simulink model "parallel_phase_voltages_per_switching_state_6"  (R2022a)
settings: Solver=FixedStepDiscrete  StartTime=0.0  StopTime=10.0  RelTol=1e-3
values from neighbouring files (symbols this model uses):
  f_c = 100000    [MPC_params.m]
  Rt = 1e-8    (= 1e-08)    [MPC_params.m]
  u_dc = 565    [MPC_params.m]
libraries: simulink x2, hdlsllib x2
(part 1 of 4)
settings Model: DataTypeOverride=Off  Creator=Andre Merx  LastModifiedBy=Andre Merx
settings SolverCC: AlgebraicLoopSolver=TrustRegion
settings DataIOCC: LimitDataPoints=on  SaveOutput=off  SaveTime=off
settings OptimizationCC: BlockReduction=off  ConditionallyExecuteInputs=off  DefaultParameterBehavior=Inlined  LifeSpan=inf
settings DebuggingCC: AlgebraicLoopMsg=error  SingleTaskRateTransMsg=error  UnconnectedInputMsg=warning  UnconnectedOutputMsg=warning  UnconnectedLineMsg=warning  AllowSymbolicDim=off  StrictBusMsg=ErrorOnBusTreatedAsVector  SFUnexpectedBacktrackingDiag=warning  SFNoUnconditionalDefaultTransitionDiag=warning  SFExecutionAtInitializationDiag=none  SFMachineParentedDataDiag=warning  ArithmeticOperatorsInVariantConditions=warning
settings HardwareCC: ProdBitPerPointer=32  ProdBitPerSizeT=32  ProdBitPerPtrDiffT=32  ProdLargestAtomicFloat=None  ProdIntDivRoundTo=Undefined  ProdEndianess=Unspecified  ProdWordSize=32  ProdHWDeviceType=ASIC/FPGA->ASIC/FPGA  ProdEqTarget=off
settings SFSimCC: SimUseLocalCustomCode=off  CustomCodeUndefinedFunction=UseInterfaceOnly
settings RTWCC: RTWUseLocalCustomCode=off
settings CodeAppCC: StateflowObjectComments=on
settings GRTTargetCC: TargetLangStandard=C89/C90 (ANSI)
settings ConfigComp: CovScope=ReferencedModels  CovMetricSettings=dw  CovSaveCumulativeToWorkspaceVar=on  CovSaveSingleToWorkspaceVar=on  CovExternalEMLEnable=off  CovSFcnEnable=off

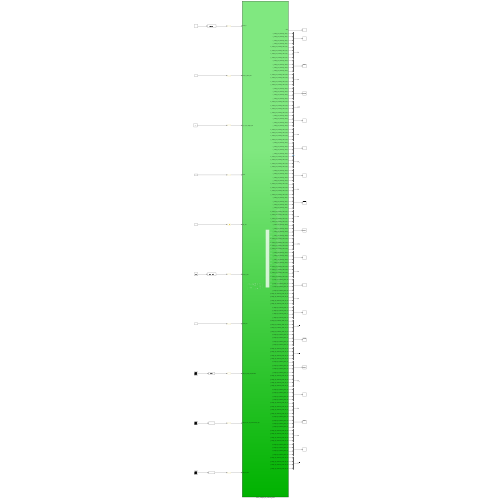
[thumbnail: Simulink's stored preview of the top-level diagram]
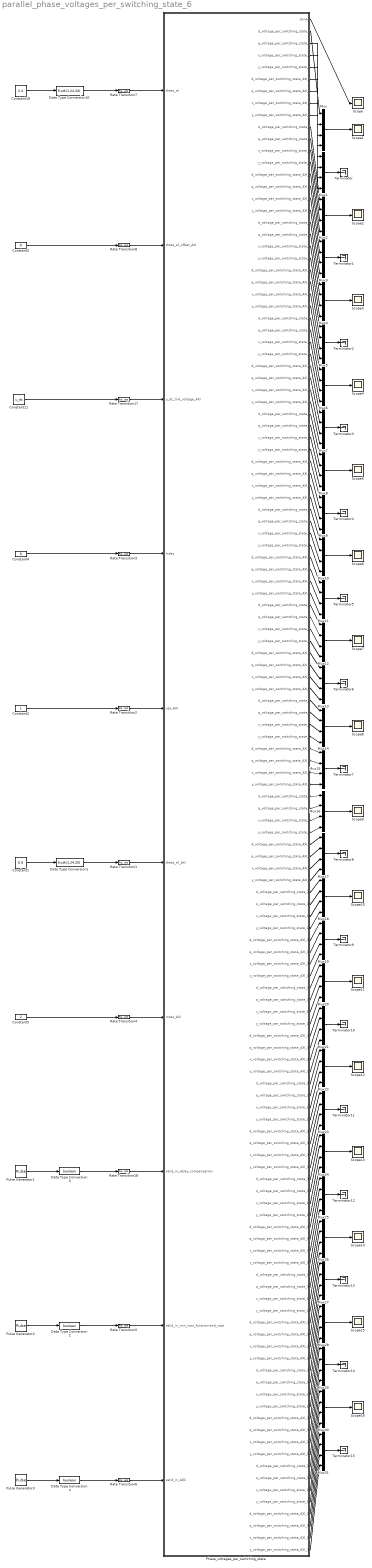
== system parallel_phase_voltages_per_switching_state_6 ==
  Constant1 : Constant  Value=0.9
  Constant11 : Constant  Value=u_dc  OutDataTypeStr=single  SampleTime=-1
  Constant18 : Constant  Value=2.4
  Constant2 : Constant  OutDataTypeStr=boolean  SampleTime=-1
  Constant3 : Constant  Value=0  OutDataTypeStr=single  SampleTime=-1
  Constant4 : Constant  Value=0  OutDataTypeStr=int32  SampleTime=-1
  Constant5 : Constant  Value=2  OutDataTypeStr=int32  SampleTime=-1
  Data Type Conversion1 : DataTypeConversion  OutDataTypeStr=fixdt(1,24,20)  SaturateOnIntegerOverflow=off  RndMeth=Floor
  Data Type Conversion10 : DataTypeConversion  OutDataTypeStr=fixdt(1,24,20)  SaturateOnIntegerOverflow=off  RndMeth=Floor
  Data Type Conversion2 : DataTypeConversion  OutDataTypeStr=boolean  SaturateOnIntegerOverflow=off  RndMeth=Floor
  Data Type Conversion3 : DataTypeConversion  OutDataTypeStr=boolean  SaturateOnIntegerOverflow=off  RndMeth=Floor
  Data Type Conversion4 : DataTypeConversion  OutDataTypeStr=boolean  SaturateOnIntegerOverflow=off  RndMeth=Floor
  Mux{,1..31} (32 alike) : Mux
  Phase_voltages_per_switching_state : Subsystem  TreatAsAtomicUnit=on
  Pulse Generator1 : DiscretePulseGenerator  PulseType=Time based  Period=1/f_c
  Pulse Generator2 : DiscretePulseGenerator  PulseType=Time based  Period=1/f_c
  Pulse Generator3 : DiscretePulseGenerator  PulseType=Time based  Period=1/f_c
  Rate Transition{1..8,17..18} (10 alike) : RateTransition  OutPortSampleTime=Rt
  Scope{,1..16} (17 alike) : Scope
  Terminator{,1..15} (16 alike) : Terminator
  wires:
  Data Type Conversion2/1 -> Rate Transition5/1
  Data Type Conversion3/1 -> Rate Transition18/1
  Rate Transition5/1 -> Phase_voltages_per_switching_state/9(valid_in_min_cost_function-and_vopt)
  Rate Transition4/1 -> Phase_voltages_per_switching_state/7(Index_AXI)
  Constant5/1 -> Rate Transition4/1
  Rate Transition6/1 -> Phase_voltages_per_switching_state/10(valid_in_ADC)
  Data Type Conversion4/1 -> Rate Transition6/1
  Pulse Generator3/1 -> Data Type Conversion4/1
  Pulse Generator2/1 -> Data Type Conversion2/1
  Rate Transition3/1 -> Phase_voltages_per_switching_state/4(Index)
  Data Type Conversion1/1 -> Rate Transition1/1
  Rate Transition18/1 -> Phase_voltages_per_switching_state/8(valid_in_delay_compensation)
  Constant18/1 -> Data Type Conversion10/1
  Rate Transition8/1 -> Phase_voltages_per_switching_state/2(theta_el_offset_AXI)
  Rate Transition1/1 -> Phase_voltages_per_switching_state/6(theta_el_AXI)
  Pulse Generator1/1 -> Data Type Conversion3/1
  Constant1/1 -> Data Type Conversion1/1
  Rate Transition7/1 -> Phase_voltages_per_switching_state/1(theta_el)
  Constant4/1 -> Rate Transition3/1
  Rate Transition17/1 -> Phase_voltages_per_switching_state/3(u_dc_link_voltage_AXI)
  Constant3/1 -> Rate Transition8/1
  Constant11/1 -> Rate Transition17/1
  Constant2/1 -> Rate Transition2/1
  Rate Transition2/1 -> Phase_voltages_per_switching_state/5(use_AXI)
  Data Type Conversion10/1 -> Rate Transition7/1
  Phase_voltages_per_switching_state/1(done) -> Scope/1
  Phase_voltages_per_switching_state/2(d_voltage_per_switching_state_1) -> Mux/1
  Phase_voltages_per_switching_state/5(y_voltage_per_switching_state_1) -> Mux/4
  Phase_voltages_per_switching_state/4(x_voltage_per_switching_state_1) -> Mux/3
  Mux/1 -> Scope1/1
  Phase_voltages_per_switching_state/3(q_voltage_per_switching_state_1) -> Mux/2
  Phase_voltages_per_switching_state/8(x_voltage_per_switching_state_AXI_1) -> Mux1/3
  Phase_voltages_per_switching_state/7(q_voltage_per_switching_state_AXI_1) -> Mux1/2
  Phase_voltages_per_switching_state/6(d_voltage_per_switching_state_AXI_1) -> Mux1/1
  Phase_voltages_per_switching_state/9(y_voltage_per_switching_state_AXI_1) -> Mux1/4
  Mux1/1 -> Terminator/1
  Phase_voltages_per_switching_state/17(y_voltage_per_switching_state_AXI_2) -> Mux3/4
  Phase_voltages_per_switching_state/12(x_voltage_per_switching_state_2) -> Mux2/3
  Mux2/1 -> Scope2/1
  Phase_voltages_per_switching_state/11(q_voltage_per_switching_state_2) -> Mux2/2
  Phase_voltages_per_switching_state/10(d_voltage_per_switching_state_2) -> Mux2/1
  Phase_voltages_per_switching_state/13(y_voltage_per_switching_state_2) -> Mux2/4
  Mux3/1 -> Terminator1/1
  Phase_voltages_per_switching_state/14(d_voltage_per_switching_state_AXI_2) -> Mux3/1
  Phase_voltages_per_switching_state/16(x_voltage_per_switching_state_AXI_2) -> Mux3/3
  Phase_voltages_per_switching_state/15(q_voltage_per_switching_state_AXI_2) -> Mux3/2
  Phase_voltages_per_switching_state/25(y_voltage_per_switching_state_AXI_3) -> Mux5/4
  Phase_voltages_per_switching_state/20(x_voltage_per_switching_state_3) -> Mux4/3
  Mux4/1 -> Scope3/1
  Phase_voltages_per_switching_state/19(q_voltage_per_switching_state_3) -> Mux4/2
  Phase_voltages_per_switching_state/18(d_voltage_per_switching_state_3) -> Mux4/1
  Phase_voltages_per_switching_state/21(y_voltage_per_switching_state_3) -> Mux4/4
  Mux5/1 -> Terminator2/1
  Phase_voltages_per_switching_state/22(d_voltage_per_switching_state_AXI_3) -> Mux5/1
  Phase_voltages_per_switching_state/24(x_voltage_per_switching_state_AXI_3) -> Mux5/3
  Phase_voltages_per_switching_state/23(q_voltage_per_switching_state_AXI_3) -> Mux5/2
  Phase_voltages_per_switching_state/33(y_voltage_per_switching_state_AXI_4) -> Mux7/4
  Phase_voltages_per_switching_state/28(x_voltage_per_switching_state_4) -> Mux6/3
  Mux6/1 -> Scope4/1
  Phase_voltages_per_switching_state/27(q_voltage_per_switching_state_4) -> Mux6/2
  Phase_voltages_per_switching_state/26(d_voltage_per_switching_state_4) -> Mux6/1
  Phase_voltages_per_switching_state/29(y_voltage_per_switching_state_4) -> Mux6/4
  Mux7/1 -> Terminator3/1
  Phase_voltages_per_switching_state/30(d_voltage_per_switching_state_AXI_4) -> Mux7/1
  Phase_voltages_per_switching_state/32(x_voltage_per_switching_state_AXI_4) -> Mux7/3
  Phase_voltages_per_switching_state/31(q_voltage_per_switching_state_AXI_4) -> Mux7/2
  Phase_voltages_per_switching_state/41(y_voltage_per_switching_state_AXI_5) -> Mux9/4
  Phase_voltages_per_switching_state/36(x_voltage_per_switching_state_5) -> Mux8/3
  Mux8/1 -> Scope5/1
  Phase_voltages_per_switching_state/35(q_voltage_per_switching_state_5) -> Mux8/2
  Phase_voltages_per_switching_state/34(d_voltage_per_switching_state_5) -> Mux8/1
  Phase_voltages_per_switching_state/37(y_voltage_per_switching_state_5) -> Mux8/4
  Mux9/1 -> Terminator4/1
  Phase_voltages_per_switching_state/38(d_voltage_per_switching_state_AXI_5) -> Mux9/1
  Phase_voltages_per_switching_state/40(x_voltage_per_switching_state_AXI_5) -> Mux9/3
  Phase_voltages_per_switching_state/39(q_voltage_per_switching_state_AXI_5) -> Mux9/2
  Phase_voltages_per_switching_state/49(y_voltage_per_switching_state_AXI_6) -> Mux11/4
  Phase_voltages_per_switching_state/44(x_voltage_per_switching_state_6) -> Mux10/3
  Mux10/1 -> Scope6/1
  Phase_voltages_per_switching_state/43(q_voltage_per_switching_state_6) -> Mux10/2
  Phase_voltages_per_switching_state/42(d_voltage_per_switching_state_6) -> Mux10/1
  Phase_voltages_per_switching_state/45(y_voltage_per_switching_state_6) -> Mux10/4
  Mux11/1 -> Terminator5/1
  Phase_voltages_per_switching_state/46(d_voltage_per_switching_state_AXI_6) -> Mux11/1
  Phase_voltages_per_switching_state/48(x_voltage_per_switching_state_AXI_6) -> Mux11/3
  Phase_voltages_per_switching_state/47(q_voltage_per_switching_state_AXI_6) -> Mux11/2
  Phase_voltages_per_switching_state/57(y_voltage_per_switching_state_AXI_7) -> Mux13/4
  Phase_voltages_per_switching_state/52(x_voltage_per_switching_state_7) -> Mux12/3
  Mux12/1 -> Scope7/1
  Phase_voltages_per_switching_state/51(q_voltage_per_switching_state_7) -> Mux12/2
  Phase_voltages_per_switching_state/50(d_voltage_per_switching_state_7) -> Mux12/1
  Phase_voltages_per_switching_state/53(y_voltage_per_switching_state_7) -> Mux12/4
  Mux13/1 -> Terminator6/1
  Phase_voltages_per_switching_state/54(d_voltage_per_switching_state_AXI_7) -> Mux13/1
  Phase_voltages_per_switching_state/56(x_voltage_per_switching_state_AXI_7) -> Mux13/3
  Phase_voltages_per_switching_state/55(q_voltage_per_switching_state_AXI_7) -> Mux13/2
  Phase_voltages_per_switching_state/65(y_voltage_per_switching_state_AXI_8) -> Mux15/4
  Phase_voltages_per_switching_state/60(x_voltage_per_switching_state_8) -> Mux14/3
  Mux14/1 -> Scope8/1
  Phase_voltages_per_switching_state/59(q_voltage_per_switching_state_8) -> Mux14/2
  Phase_voltages_per_switching_state/58(d_voltage_per_switching_state_8) -> Mux14/1
  Phase_voltages_per_switching_state/61(y_voltage_per_switching_state_8) -> Mux14/4
  Mux15/1 -> Terminator7/1
  Phase_voltages_per_switching_state/62(d_voltage_per_switching_state_AXI_8) -> Mux15/1
  Phase_voltages_per_switching_state/64(x_voltage_per_switching_state_AXI_8) -> Mux15/3
  Phase_voltages_per_switching_state/63(q_voltage_per_switching_state_AXI_8) -> Mux15/2
  Phase_voltages_per_switching_state/73(y_voltage_per_switching_state_AXI_9) -> Mux17/4
  Phase_voltages_per_switching_state/68(x_voltage_per_switching_state_9) -> Mux16/3
  Mux16/1 -> Scope9/1
  Phase_voltages_per_switching_state/67(q_voltage_per_switching_state_9) -> Mux16/2
  Phase_voltages_per_switching_state/66(d_voltage_per_switching_state_9) -> Mux16/1
  Phase_voltages_per_switching_state/69(y_voltage_per_switching_state_9) -> Mux16/4
  Mux17/1 -> Terminator8/1
  Phase_voltages_per_switching_state/70(d_voltage_per_switching_state_AXI_9) -> Mux17/1
  Phase_voltages_per_switching_state/72(x_voltage_per_switching_state_AXI_9) -> Mux17/3
  Phase_voltages_per_switching_state/71(q_voltage_per_switching_state_AXI_9) -> Mux17/2
  Phase_voltages_per_switching_state/81(y_voltage_per_switching_state_AXI_10) -> Mux19/4
  Phase_voltages_per_switching_state/76(x_voltage_per_switching_state_10) -> Mux18/3
  Mux18/1 -> Scope10/1
  Phase_voltages_per_switching_state/75(q_voltage_per_switching_state_10) -> Mux18/2
  Phase_voltages_per_switching_state/74(d_voltage_per_switching_state_10) -> Mux18/1
  Phase_voltages_per_switching_state/77(y_voltage_per_switching_state_10) -> Mux18/4
  Mux19/1 -> Terminator9/1
  Phase_voltages_per_switching_state/78(d_voltage_per_switching_state_AXI_10) -> Mux19/1
  Phase_voltages_per_switching_state/80(x_voltage_per_switching_state_AXI_10) -> Mux19/3
  Phase_voltages_per_switching_state/79(q_voltage_per_switching_state_AXI_10) -> Mux19/2
  Phase_voltages_per_switching_state/89(y_voltage_per_switching_state_AXI_11) -> Mux21/4
  Phase_voltages_per_switching_state/84(x_voltage_per_switching_state_11) -> Mux20/3
  Mux20/1 -> Scope11/1
  Phase_voltages_per_switching_state/83(q_voltage_per_switching_state_11) -> Mux20/2
  Phase_voltages_per_switching_state/82(d_voltage_per_switching_state_11) -> Mux20/1
  Phase_voltages_per_switching_state/85(y_voltage_per_switching_state_11) -> Mux20/4
  Mux21/1 -> Terminator10/1
  Phase_voltages_per_switching_state/86(d_voltage_per_switching_state_AXI_11) -> Mux21/1
  Phase_voltages_per_switching_state/88(x_voltage_per_switching_state_AXI_11) -> Mux21/3
  Phase_voltages_per_switching_state/87(q_voltage_per_switching_state_AXI_11) -> Mux21/2
  Phase_voltages_per_switching_state/97(y_voltage_per_switching_state_AXI_12) -> Mux23/4
  Phase_voltages_per_switching_state/92(x_voltage_per_switching_state_12) -> Mux22/3
  Mux22/1 -> Scope12/1
  Phase_voltages_per_switching_state/91(q_voltage_per_switching_state_12) -> Mux22/2
  Phase_voltages_per_switching_state/90(d_voltage_per_switching_state_12) -> Mux22/1
  Phase_voltages_per_switching_state/93(y_voltage_per_switching_state_12) -> Mux22/4
  Mux23/1 -> Terminator11/1
  Phase_voltages_per_switching_state/94(d_voltage_per_switching_state_AXI_12) -> Mux23/1
  Phase_voltages_per_switching_state/96(x_voltage_per_switching_state_AXI_12) -> Mux23/3
  Phase_voltages_per_switching_state/95(q_voltage_per_switching_state_AXI_12) -> Mux23/2
  Phase_voltages_per_switching_state/105(y_voltage_per_switching_state_AXI_13) -> Mux25/4
  Phase_voltages_per_switching_state/100(x_voltage_per_switching_state_13) -> Mux24/3
  Mux24/1 -> Scope13/1
  Phase_voltages_per_switching_state/99(q_voltage_per_switching_state_13) -> Mux24/2
  Phase_voltages_per_switching_state/98(d_voltage_per_switching_state_13) -> Mux24/1
  Phase_voltages_per_switching_state/101(y_voltage_per_switching_state_13) -> Mux24/4
  Mux25/1 -> Terminator12/1
  Phase_voltages_per_switching_state/102(d_voltage_per_switching_state_AXI_13) -> Mux25/1
  Phase_voltages_per_switching_state/104(x_voltage_per_switching_state_AXI_13) -> Mux25/3
  Phase_voltages_per_switching_state/103(q_voltage_per_switching_state_AXI_13) -> Mux25/2
  Phase_voltages_per_switching_state/113(y_voltage_per_switching_state_AXI_14) -> Mux27/4
  Phase_voltages_per_switching_state/108(x_voltage_per_switching_state_14) -> Mux26/3
  Mux26/1 -> Scope14/1
  Phase_voltages_per_switching_state/107(q_voltage_per_switching_state_14) -> Mux26/2
  Phase_voltages_per_switching_state/106(d_voltage_per_switching_state_14) -> Mux26/1
  Phase_voltages_per_switching_state/109(y_voltage_per_switching_state_14) -> Mux26/4
  Mux27/1 -> Terminator13/1
  Phase_voltages_per_switching_state/110(d_voltage_per_switching_state_AXI_14) -> Mux27/1
  Phase_voltages_per_switching_state/112(x_voltage_per_switching_state_AXI_14) -> Mux27/3
  Phase_voltages_per_switching_state/111(q_voltage_per_switching_state_AXI_14) -> Mux27/2
  Phase_voltages_per_switching_state/121(y_voltage_per_switching_state_AXI_15) -> Mux29/4
  Phase_voltages_per_switching_state/116(x_voltage_per_switching_state_15) -> Mux28/3
  Mux28/1 -> Scope15/1
  Phase_voltages_per_switching_state/115(q_voltage_per_switching_state_15) -> Mux28/2
  Phase_voltages_per_switching_state/114(d_voltage_per_switching_state_15) -> Mux28/1
  Phase_voltages_per_switching_state/117(y_voltage_per_switching_state_15) -> Mux28/4
  Mux29/1 -> Terminator14/1
  Phase_voltages_per_switching_state/118(d_voltage_per_switching_state_AXI_15) -> Mux29/1
  Phase_voltages_per_switching_state/120(x_voltage_per_switching_state_AXI_15) -> Mux29/3
  Phase_voltages_per_switching_state/119(q_voltage_per_switching_state_AXI_15) -> Mux29/2
  Phase_voltages_per_switching_state/129(y_voltage_per_switching_state_AXI_16) -> Mux31/4
  Phase_voltages_per_switching_state/124(x_voltage_per_switching_state_16) -> Mux30/3
  Mux30/1 -> Scope16/1
  Phase_voltages_per_switching_state/123(q_voltage_per_switching_state_16) -> Mux30/2
  Phase_voltages_per_switching_state/122(d_voltage_per_switching_state_16) -> Mux30/1
  Phase_voltages_per_switching_state/125(y_voltage_per_switching_state_16) -> Mux30/4
  Mux31/1 -> Terminator15/1
  Phase_voltages_per_switching_state/126(d_voltage_per_switching_state_AXI_16) -> Mux31/1
  Phase_voltages_per_switching_state/128(x_voltage_per_switching_state_AXI_16) -> Mux31/3
  Phase_voltages_per_switching_state/127(q_voltage_per_switching_state_AXI_16) -> Mux31/2

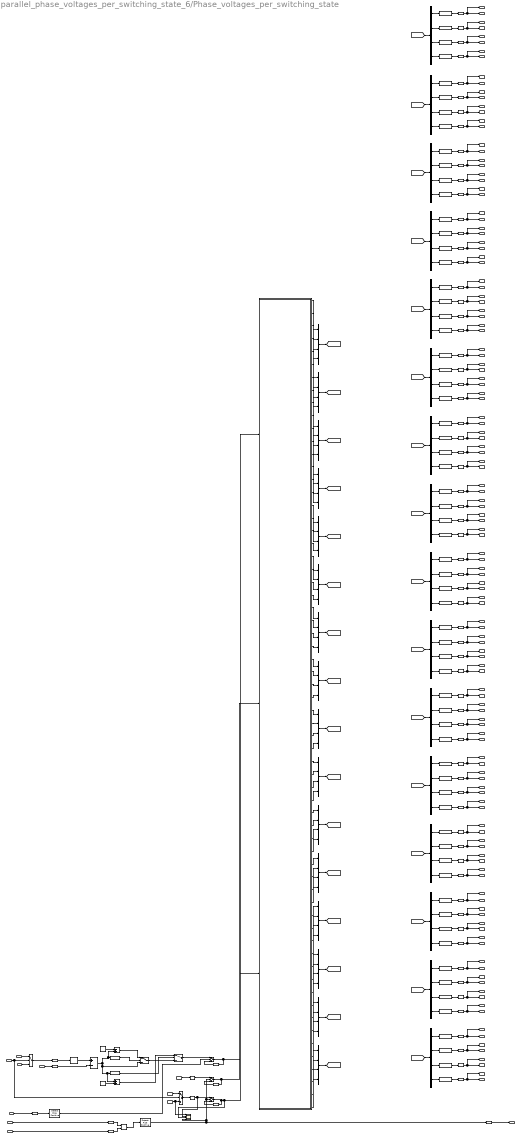
== system parallel_phase_voltages_per_switching_state_6/Phase_voltages_per_switching_state ==
  theta_el : Inport
  theta_el_offset_AXI : Inport  Port=2
  u_dc_link_voltage_AXI : Inport  Port=3
  Index : Inport  Port=4
  use_AXI : Inport  Port=5
  theta_el_AXI : Inport  Port=6
  Index_AXI : Inport  Port=7
  valid_in_delay_compensation : Inport  Port=8
  valid_in_min_cost_function-and_vopt : Inport  Port=9
  valid_in_ADC : Inport  Port=10
  Add1 : Sum  Inputs=+-  OutDataTypeStr=Inherit: Same as accumulator
  Add2 : Sum  Inputs=-+  OutDataTypeStr=Inherit: Same as first input
  Add3 : Sum  OutDataTypeStr=Inherit: Same as first input
  Compare Limit_High : simulink/Logic and Bit Operations/Compare To Constant  relop=>=  const=2*pi  OutDataTypeStr=boolean
  Compare Limit_Low : simulink/Logic and Bit Operations/Compare To Constant  relop=<  const=0  OutDataTypeStr=boolean
  Constant : Constant  Value=2*pi  OutDataTypeStr=single  SampleTime=Rt
  Constant1 : Constant  Value=2*pi  OutDataTypeStr=single  SampleTime=Rt
  Data Type Conversion{1..5,7..65} (64 alike) : DataTypeConversion  OutDataTypeStr=fixdt(1,24,11)  SaturateOnIntegerOverflow=off  RndMeth=Floor
  Data Type Conversion6 : DataTypeConversion  OutDataTypeStr=single  RndMeth=Nearest  SaturateOnIntegerOverflow=off
  Delay{1..10,13..75} (73 alike) : Delay  DelayLength=1
  Delay11 : Delay  DelayLength=3
  Delay12 : Delay  DelayLength=3
  Demux{,1..15} (16 alike) : Demux
  Detect Rise Positive : hdlsllib/Logic and Bit Operations/Detect Rise Positive  vinit=0  OutDataTypeStr=boolean
      settings: SourceProductBaseCode=SL
  Detect Rise Positive1 : hdlsllib/Logic and Bit Operations/Detect Rise Positive  vinit=0  OutDataTypeStr=boolean
      settings: SourceProductBaseCode=SL
  Logical Operator : Logic  Operator=OR  AllPortsSameDT=off  OutDataTypeStr=boolean
  Mux{,1..15} (16 alike) : Mux
  Scope2 : Scope  NumInputPorts=4
  Subsystem : Subsystem
  Switch_Limit_High : Switch  Criteria=u2 > Threshold  OutDataTypeStr=single  SaturateOnIntegerOverflow=off  InputSameDT=off
  Switch_Limit_Low : Switch  Criteria=u2 > Threshold  OutDataTypeStr=single  SaturateOnIntegerOverflow=off  InputSameDT=off
  Switch_on1 : Switch  Threshold=1  OutDataTypeStr=single  RndMeth=Simplest  SaturateOnIntegerOverflow=off  InputSameDT=off
  Switch_on13 : Switch  Threshold=1  OutDataTypeStr=single  RndMeth=Simplest  SaturateOnIntegerOverflow=off  InputSameDT=off
  Switch_on2 : Switch  Threshold=1  OutDataTypeStr=Inherit: Inherit via back propagation  RndMeth=Simplest  SaturateOnIntegerOverflow=off  InputSameDT=off
  Switch_on3 : Switch  Threshold=1  OutDataTypeStr=Inherit: Inherit via back propagation  RndMeth=Simplest  SaturateOnIntegerOverflow=off  InputSameDT=off
  Switch_on6 : Switch  Threshold=1  OutDataTypeStr=Inherit: Inherit via back propagation  RndMeth=Simplest  SaturateOnIntegerOverflow=off  InputSameDT=off
  done : Outport
  d_voltage_per_switching_state_1 : Outport  Port=2
  q_voltage_per_switching_state_1 : Outport  Port=3
  x_voltage_per_switching_state_1 : Outport  Port=4
  y_voltage_per_switching_state_1 : Outport  Port=5
  d_voltage_per_switching_state_AXI_1 : Outport  Port=6
  q_voltage_per_switching_state_AXI_1 : Outport  Port=7
  x_voltage_per_switching_state_AXI_1 : Outport  Port=8
  y_voltage_per_switching_state_AXI_1 : Outport  Port=9
  d_voltage_per_switching_state_2 : Outport  Port=10
  q_voltage_per_switching_state_2 : Outport  Port=11
  x_voltage_per_switching_state_2 : Outport  Port=12
  y_voltage_per_switching_state_2 : Outport  Port=13
  d_voltage_per_switching_state_AXI_2 : Outport  Port=14
  q_voltage_per_switching_state_AXI_2 : Outport  Port=15
  x_voltage_per_switching_state_AXI_2 : Outport  Port=16
  y_voltage_per_switching_state_AXI_2 : Outport  Port=17
  d_voltage_per_switching_state_3 : Outport  Port=18
  q_voltage_per_switching_state_3 : Outport  Port=19
  x_voltage_per_switching_state_3 : Outport  Port=20
  y_voltage_per_switching_state_3 : Outport  Port=21
  d_voltage_per_switching_state_AXI_3 : Outport  Port=22
  q_voltage_per_switching_state_AXI_3 : Outport  Port=23
  x_voltage_per_switching_state_AXI_3 : Outport  Port=24
  y_voltage_per_switching_state_AXI_3 : Outport  Port=25
  d_voltage_per_switching_state_4 : Outport  Port=26
  q_voltage_per_switching_state_4 : Outport  Port=27
  x_voltage_per_switching_state_4 : Outport  Port=28
  y_voltage_per_switching_state_4 : Outport  Port=29
  d_voltage_per_switching_state_AXI_4 : Outport  Port=30
  q_voltage_per_switching_state_AXI_4 : Outport  Port=31
  x_voltage_per_switching_state_AXI_4 : Outport  Port=32
  y_voltage_per_switching_state_AXI_4 : Outport  Port=33
  d_voltage_per_switching_state_5 : Outport  Port=34
  q_voltage_per_switching_state_5 : Outport  Port=35
  x_voltage_per_switching_state_5 : Outport  Port=36
  y_voltage_per_switching_state_5 : Outport  Port=37
  d_voltage_per_switching_state_AXI_5 : Outport  Port=38
  q_voltage_per_switching_state_AXI_5 : Outport  Port=39
  x_voltage_per_switching_state_AXI_5 : Outport  Port=40
  y_voltage_per_switching_state_AXI_5 : Outport  Port=41
  d_voltage_per_switching_state_6 : Outport  Port=42
  q_voltage_per_switching_state_6 : Outport  Port=43
  x_voltage_per_switching_state_6 : Outport  Port=44
  y_voltage_per_switching_state_6 : Outport  Port=45
  d_voltage_per_switching_state_AXI_6 : Outport  Port=46
  q_voltage_per_switching_state_AXI_6 : Outport  Port=47
  x_voltage_per_switching_state_AXI_6 : Outport  Port=48
  y_voltage_per_switching_state_AXI_6 : Outport  Port=49
  d_voltage_per_switching_state_7 : Outport  Port=50
  q_voltage_per_switching_state_7 : Outport  Port=51
  x_voltage_per_switching_state_7 : Outport  Port=52
  y_voltage_per_switching_state_7 : Outport  Port=53
  d_voltage_per_switching_state_AXI_7 : Outport  Port=54
  q_voltage_per_switching_state_AXI_7 : Outport  Port=55
  x_voltage_per_switching_state_AXI_7 : Outport  Port=56
  y_voltage_per_switching_state_AXI_7 : Outport  Port=57
  d_voltage_per_switching_state_8 : Outport  Port=58
  q_voltage_per_switching_state_8 : Outport  Port=59
  x_voltage_per_switching_state_8 : Outport  Port=60
  y_voltage_per_switching_state_8 : Outport  Port=61
  d_voltage_per_switching_state_AXI_8 : Outport  Port=62
  q_voltage_per_switching_state_AXI_8 : Outport  Port=63
  x_voltage_per_switching_state_AXI_8 : Outport  Port=64
  y_voltage_per_switching_state_AXI_8 : Outport  Port=65
  d_voltage_per_switching_state_9 : Outport  Port=66
  q_voltage_per_switching_state_9 : Outport  Port=67
  x_voltage_per_switching_state_9 : Outport  Port=68
  y_voltage_per_switching_state_9 : Outport  Port=69
  d_voltage_per_switching_state_AXI_9 : Outport  Port=70
  q_voltage_per_switching_state_AXI_9 : Outport  Port=71
  x_voltage_per_switching_state_AXI_9 : Outport  Port=72
  y_voltage_per_switching_state_AXI_9 : Outport  Port=73
  d_voltage_per_switching_state_10 : Outport  Port=74
  q_voltage_per_switching_state_10 : Outport  Port=75
  x_voltage_per_switching_state_10 : Outport  Port=76
  y_voltage_per_switching_state_10 : Outport  Port=77
  d_voltage_per_switching_state_AXI_10 : Outport  Port=78
  q_voltage_per_switching_state_AXI_10 : Outport  Port=79
  x_voltage_per_switching_state_AXI_10 : Outport  Port=80
  y_voltage_per_switching_state_AXI_10 : Outport  Port=81
  d_voltage_per_switching_state_11 : Outport  Port=82
  q_voltage_per_switching_state_11 : Outport  Port=83
  x_voltage_per_switching_state_11 : Outport  Port=84
  y_voltage_per_switching_state_11 : Outport  Port=85
  d_voltage_per_switching_state_AXI_11 : Outport  Port=86
  q_voltage_per_switching_state_AXI_11 : Outport  Port=87
  x_voltage_per_switching_state_AXI_11 : Outport  Port=88
  y_voltage_per_switching_state_AXI_11 : Outport  Port=89
  d_voltage_per_switching_state_12 : Outport  Port=90
  q_voltage_per_switching_state_12 : Outport  Port=91
  x_voltage_per_switching_state_12 : Outport  Port=92
  y_voltage_per_switching_state_12 : Outport  Port=93
  d_voltage_per_switching_state_AXI_12 : Outport  Port=94
  q_voltage_per_switching_state_AXI_12 : Outport  Port=95
  x_voltage_per_switching_state_AXI_12 : Outport  Port=96
  y_voltage_per_switching_state_AXI_12 : Outport  Port=97
  d_voltage_per_switching_state_13 : Outport  Port=98
  q_voltage_per_switching_state_13 : Outport  Port=99
  x_voltage_per_switching_state_13 : Outport  Port=100
  y_voltage_per_switching_state_13 : Outport  Port=101
  d_voltage_per_switching_state_AXI_13 : Outport  Port=102
  q_voltage_per_switching_state_AXI_13 : Outport  Port=103
  x_voltage_per_switching_state_AXI_13 : Outport  Port=104
  y_voltage_per_switching_state_AXI_13 : Outport  Port=105
  d_voltage_per_switching_state_14 : Outport  Port=106
  q_voltage_per_switching_state_14 : Outport  Port=107
  x_voltage_per_switching_state_14 : Outport  Port=108
  y_voltage_per_switching_state_14 : Outport  Port=109
  d_voltage_per_switching_state_AXI_14 : Outport  Port=110
  q_voltage_per_switching_state_AXI_14 : Outport  Port=111
  x_voltage_per_switching_state_AXI_14 : Outport  Port=112
  y_voltage_per_switching_state_AXI_14 : Outport  Port=113
  d_voltage_per_switching_state_15 : Outport  Port=114
  q_voltage_per_switching_state_15 : Outport  Port=115
  x_voltage_per_switching_state_15 : Outport  Port=116
  y_voltage_per_switching_state_15 : Outport  Port=117
  d_voltage_per_switching_state_AXI_15 : Outport  Port=118
  q_voltage_per_switching_state_AXI_15 : Outport  Port=119
  x_voltage_per_switching_state_AXI_15 : Outport  Port=120
  y_voltage_per_switching_state_AXI_15 : Outport  Port=121
  d_voltage_per_switching_state_16 : Outport  Port=122
  q_voltage_per_switching_state_16 : Outport  Port=123
  x_voltage_per_switching_state_16 : Outport  Port=124
  y_voltage_per_switching_state_16 : Outport  Port=125
  d_voltage_per_switching_state_AXI_16 : Outport  Port=126
  q_voltage_per_switching_state_AXI_16 : Outport  Port=127
  x_voltage_per_switching_state_AXI_16 : Outport  Port=128
  y_voltage_per_switching_state_AXI_16 : Outport  Port=129
  wires:
  Delay8/1 -> Data Type Conversion6/1
  Compare Limit_High/1 -> Switch_Limit_High/2
  Delay14/1 -> Switch_on3/3
  Delay7/1 -> y_voltage_per_switching_state_16/1, y_voltage_per_switching_state_AXI_16/1
  Delay13/1 -> Switch_on13/3
  Switch_on13/1 -> Subsystem/1(theta_el_with_offset15), Delay13/1
  u_dc_link_voltage_AXI/1 -> Delay10/1  "End_Cycle"
  theta_el_offset_AXI/1 -> Delay9/1
  Delay6/1 -> x_voltage_per_switching_state_16/1, x_voltage_per_switching_state_AXI_16/1
  Switch_Limit_High/1 -> Switch_Limit_Low/3
  Constant/1 -> Add2/1
  Delay10/1 -> Switch_on1/1
  Delay12/1 -> Logical Operator/1
  Delay9/1 -> Add1/2
  Add3/1 -> Switch_Limit_Low/1
  Delay5/1 -> q_voltage_per_switching_state_16/1, q_voltage_per_switching_state_AXI_16/1
  Data Type Conversion6/1 -> Add1/1  "End_Cycle"
  Switch_Limit_Low/1 -> Switch_on13/1  "End_Cycle"
  Add1/1 -> Switch_Limit_High/3, Add3/1, Compare Limit_Low/1, Add2/2, Compare Limit_High/1
  valid_in_delay_compensation/1 -> Delay12/1
  Switch_on1/1 -> Subsystem/2(u_dc_link_voltage15), Delay1/1
  Detect Rise Positive1/1 -> Switch_on3/2, Switch_on1/2, Scope2/4, Delay3/1  "End_Cycle"
  Compare Limit_Low/1 -> Switch_Limit_Low/2
  Delay1/1 -> Switch_on1/3
  Constant1/1 -> Add3/2
  Delay3/1 -> done/1
  Delay4/1 -> d_voltage_per_switching_state_16/1, d_voltage_per_switching_state_AXI_16/1
  Add2/1 -> Switch_Limit_High/1
  theta_el/1 -> Switch_on2/3
  Switch_on2/1 -> Delay8/1
  theta_el_AXI/1 -> Switch_on2/1
  use_AXI/1 -> Switch_on6/2, Switch_on2/2
  Data Type Conversion10/1 -> Delay4/1
  Data Type Conversion1/1 -> Delay5/1
  Data Type Conversion2/1 -> Delay6/1
  Data Type Conversion3/1 -> Delay7/1
  Delay2/1 -> Scope2/2, Switch_on3/1
  Switch_on6/1 -> Delay2/1
  Index/1 -> Scope2/1, Switch_on6/3  "End_Cycle"
  Index_AXI/1 -> Switch_on6/1  "End_Cycle"
  valid_in_min_cost_function-and_vopt/1 -> Delay11/1
  Logical Operator/1 -> Detect Rise Positive1/1
  Delay11/1 -> Logical Operator/2
  Switch_on3/1 -> Delay14/1, Subsystem/3(Index 15), Scope2/3
  valid_in_ADC/1 -> Delay21/1
  Detect Rise Positive/1 -> Switch_on13/2  "End_Cycle"
  Delay21/1 -> Detect Rise Positive/1
  Subsystem/61(d_voltage_per_switching_state15) -> Mux/1
  Subsystem/62(q_voltage_per_switching_state15) -> Mux/2
  Subsystem/63(x_voltage_per_switching_state15) -> Mux/3
  Subsystem/64(y_voltage_per_switching_state15) -> Mux/4
  Mux/1 -> [voltage_16]
  Demux/3 -> Data Type Conversion2/1
  Demux/1 -> Data Type Conversion10/1
  Demux/2 -> Data Type Conversion1/1
  Demux/4 -> Data Type Conversion3/1
  [voltage_16] -> Demux/1
  Demux1/4 -> Data Type Conversion8/1
  Delay18/1 -> y_voltage_per_switching_state_1/1, y_voltage_per_switching_state_AXI_1/1
  Delay16/1 -> q_voltage_per_switching_state_1/1, q_voltage_per_switching_state_AXI_1/1
  Delay17/1 -> x_voltage_per_switching_state_1/1, x_voltage_per_switching_state_AXI_1/1
  [voltage_1] -> Demux1/1
  Demux1/3 -> Data Type Conversion7/1
  Demux1/1 -> Data Type Conversion5/1
  Data Type Conversion7/1 -> Delay17/1
  Data Type Conversion4/1 -> Delay16/1
  Data Type Conversion8/1 -> Delay18/1
  Delay15/1 -> d_voltage_per_switching_state_1/1, d_voltage_per_switching_state_AXI_1/1
  Demux1/2 -> Data Type Conversion4/1
  Data Type Conversion5/1 -> Delay15/1
  Mux1/1 -> [voltage_1]
  Subsystem/1(d_voltage_per_switching_state) -> Mux1/1
  Subsystem/2(q_voltage_per_switching_state) -> Mux1/2
  Subsystem/4(y_voltage_per_switching_state) -> Mux1/4
  Subsystem/3(x_voltage_per_switching_state) -> Mux1/3
  Delay23/1 -> y_voltage_per_switching_state_2/1, y_voltage_per_switching_state_AXI_2/1
  Data Type Conversion12/1 -> Delay22/1
  Data Type Conversion13/1 -> Delay23/1
  Demux2/2 -> Data Type Conversion9/1
  Demux2/4 -> Data Type Conversion13/1
  Data Type Conversion11/1 -> Delay19/1
  Delay19/1 -> d_voltage_per_switching_state_2/1, d_voltage_per_switching_state_AXI_2/1
  Data Type Conversion9/1 -> Delay20/1
  [voltage_2] -> Demux2/1
  Demux2/1 -> Data Type Conversion11/1
  Demux2/3 -> Data Type Conversion12/1
  Delay22/1 -> x_voltage_per_switching_state_2/1, x_voltage_per_switching_state_AXI_2/1
  Delay20/1 -> q_voltage_per_switching_state_2/1, q_voltage_per_switching_state_AXI_2/1
  Mux2/1 -> [voltage_2]
  Subsystem/7(x_voltage_per_switching_state1) -> Mux2/3
  Subsystem/5(d_voltage_per_switching_state1) -> Mux2/1
  Subsystem/6(q_voltage_per_switching_state1) -> Mux2/2
  Subsystem/8(y_voltage_per_switching_state1) -> Mux2/4
  Delay26/1 -> x_voltage_per_switching_state_3/1, x_voltage_per_switching_state_AXI_3/1
  Delay25/1 -> q_voltage_per_switching_state_3/1, q_voltage_per_switching_state_AXI_3/1
  Demux3/1 -> Data Type Conversion14/1
  Demux3/3 -> Data Type Conversion15/1
  [voltage_3] -> Demux3/1
  Demux3/4 -> Data Type Conversion16/1
  Demux3/2 -> Data Type Conversion17/1
  Data Type Conversion17/1 -> Delay25/1
  Delay24/1 -> d_voltage_per_switching_state_3/1, d_voltage_per_switching_state_AXI_3/1
  Data Type Conversion15/1 -> Delay26/1
  Delay27/1 -> y_voltage_per_switching_state_3/1, y_voltage_per_switching_state_AXI_3/1
  Data Type Conversion14/1 -> Delay24/1
  Data Type Conversion16/1 -> Delay27/1
  Mux3/1 -> [voltage_3]
  Subsystem/12(y_voltage_per_switching_state2) -> Mux3/4
  Subsystem/9(d_voltage_per_switching_state2) -> Mux3/1
  Subsystem/10(q_voltage_per_switching_state2) -> Mux3/2
  Subsystem/11(x_voltage_per_switching_state2) -> Mux3/3
  Data Type Conversion18/1 -> Delay28/1
  Delay28/1 -> d_voltage_per_switching_state_4/1, d_voltage_per_switching_state_AXI_4/1
  Data Type Conversion20/1 -> Delay31/1
  Delay31/1 -> y_voltage_per_switching_state_4/1, y_voltage_per_switching_state_AXI_4/1
  Demux4/4 -> Data Type Conversion20/1
  Delay30/1 -> x_voltage_per_switching_state_4/1, x_voltage_per_switching_state_AXI_4/1
  Demux4/1 -> Data Type Conversion18/1
  Demux4/2 -> Data Type Conversion21/1
  Data Type Conversion21/1 -> Delay29/1
  [voltage_4] -> Demux4/1
  Demux4/3 -> Data Type Conversion19/1
  Delay29/1 -> q_voltage_per_switching_state_4/1, q_voltage_per_switching_state_AXI_4/1
  Data Type Conversion19/1 -> Delay30/1
  Subsystem/13(d_voltage_per_switching_state3) -> Mux4/1
  Mux4/1 -> [voltage_4]
  Subsystem/15(x_voltage_per_switching_state3) -> Mux4/3
  Subsystem/16(y_voltage_per_switching_state3) -> Mux4/4
  Subsystem/14(q_voltage_per_switching_state3) -> Mux4/2
  Demux5/1 -> Data Type Conversion22/1
  [voltage_5] -> Demux5/1
  Data Type Conversion25/1 -> Delay33/1
  Delay33/1 -> q_voltage_per_switching_state_5/1, q_voltage_per_switching_state_AXI_5/1
  Delay34/1 -> x_voltage_per_switching_state_5/1, x_voltage_per_switching_state_AXI_5/1
  Demux5/2 -> Data Type Conversion25/1
  Demux5/3 -> Data Type Conversion23/1
  Data Type Conversion23/1 -> Delay34/1
  Delay35/1 -> y_voltage_per_switching_state_5/1, y_voltage_per_switching_state_AXI_5/1
  Data Type Conversion22/1 -> Delay32/1
  Delay32/1 -> d_voltage_per_switching_state_5/1, d_voltage_per_switching_state_AXI_5/1
  Data Type Conversion24/1 -> Delay35/1
  Demux5/4 -> Data Type Conversion24/1
  Mux5/1 -> [voltage_5]
  Subsystem/19(x_voltage_per_switching_state4) -> Mux5/3
  Subsystem/18(q_voltage_per_switching_state4) -> Mux5/2
  Subsystem/17(d_voltage_per_switching_state4) -> Mux5/1
  Subsystem/20(y_voltage_per_switching_state4) -> Mux5/4
  Data Type Conversion29/1 -> Delay37/1
  Data Type Conversion27/1 -> Delay38/1
  Demux6/2 -> Data Type Conversion29/1
  Delay37/1 -> q_voltage_per_switching_state_6/1, q_voltage_per_switching_state_AXI_6/1
  Demux6/3 -> Data Type Conversion27/1
  Demux6/1 -> Data Type Conversion26/1
  Demux6/4 -> Data Type Conversion28/1
  Delay38/1 -> x_voltage_per_switching_state_6/1, x_voltage_per_switching_state_AXI_6/1
  Data Type Conversion26/1 -> Delay36/1
  Delay36/1 -> d_voltage_per_switching_state_6/1, d_voltage_per_switching_state_AXI_6/1
  Data Type Conversion28/1 -> Delay39/1
  [voltage_6] -> Demux6/1
  Delay39/1 -> y_voltage_per_switching_state_6/1, y_voltage_per_switching_state_AXI_6/1
  Subsystem/23(x_voltage_per_switching_state5) -> Mux6/3
  Subsystem/21(d_voltage_per_switching_state5) -> Mux6/1
  Subsystem/22(q_voltage_per_switching_state5) -> Mux6/2
  Subsystem/24(y_voltage_per_switching_state5) -> Mux6/4
  Mux6/1 -> [voltage_6]
  Delay43/1 -> y_voltage_per_switching_state_7/1, y_voltage_per_switching_state_AXI_7/1
  Delay40/1 -> d_voltage_per_switching_state_7/1, d_voltage_per_switching_state_AXI_7/1
  [voltage_7] -> Demux7/1
  Delay42/1 -> x_voltage_per_switching_state_7/1, x_voltage_per_switching_state_AXI_7/1
  Demux7/1 -> Data Type Conversion30/1
  Demux7/4 -> Data Type Conversion32/1
  Data Type Conversion32/1 -> Delay43/1
  Data Type Conversion31/1 -> Delay42/1
  Data Type Conversion30/1 -> Delay40/1
  Delay41/1 -> q_voltage_per_switching_state_7/1, q_voltage_per_switching_state_AXI_7/1
  Demux7/3 -> Data Type Conversion31/1
  Data Type Conversion33/1 -> Delay41/1
  Demux7/2 -> Data Type Conversion33/1
  Subsystem/25(d_voltage_per_switching_state6) -> Mux7/1
  Mux7/1 -> [voltage_7]
  Subsystem/28(y_voltage_per_switching_state6) -> Mux7/4
  Subsystem/27(x_voltage_per_switching_state6) -> Mux7/3
  Subsystem/26(q_voltage_per_switching_state6) -> Mux7/2
  Data Type Conversion37/1 -> Delay45/1
  Demux8/3 -> Data Type Conversion35/1
  Delay45/1 -> q_voltage_per_switching_state_8/1, q_voltage_per_switching_state_AXI_8/1
  Data Type Conversion35/1 -> Delay46/1
  Demux8/4 -> Data Type Conversion36/1
  Data Type Conversion36/1 -> Delay47/1
  Data Type Conversion34/1 -> Delay44/1
  Delay46/1 -> x_voltage_per_switching_state_8/1, x_voltage_per_switching_state_AXI_8/1
  [voltage_8] -> Demux8/1
  Delay47/1 -> y_voltage_per_switching_state_8/1, y_voltage_per_switching_state_AXI_8/1
  Demux8/1 -> Data Type Conversion34/1
  Delay44/1 -> d_voltage_per_switching_state_8/1, d_voltage_per_switching_state_AXI_8/1
  Demux8/2 -> Data Type Conversion37/1
  Mux8/1 -> [voltage_8]
  Subsystem/29(d_voltage_per_switching_state7) -> Mux8/1
  Subsystem/32(y_voltage_per_switching_state7) -> Mux8/4
  Subsystem/30(q_voltage_per_switching_state7) -> Mux8/2
  Subsystem/31(x_voltage_per_switching_state7) -> Mux8/3
  Data Type Conversion40/1 -> Delay51/1
  Data Type Conversion38/1 -> Delay48/1
  Demux9/4 -> Data Type Conversion40/1
  Demux9/3 -> Data Type Conversion39/1
  Data Type Conversion41/1 -> Delay49/1
  Delay49/1 -> q_voltage_per_switching_state_9/1, q_voltage_per_switching_state_AXI_9/1
  Data Type Conversion39/1 -> Delay50/1
  Demux9/2 -> Data Type Conversion41/1
  Delay51/1 -> y_voltage_per_switching_state_9/1, y_voltage_per_switching_state_AXI_9/1
  Delay50/1 -> x_voltage_per_switching_state_9/1, x_voltage_per_switching_state_AXI_9/1
  Demux9/1 -> Data Type Conversion38/1
  [voltage_9] -> Demux9/1
  Delay48/1 -> d_voltage_per_switching_state_9/1, d_voltage_per_switching_state_AXI_9/1
  Subsystem/36(y_voltage_per_switching_state8) -> Mux9/4
  Subsystem/33(d_voltage_per_switching_state8) -> Mux9/1
  Subsystem/34(q_voltage_per_switching_state8) -> Mux9/2
  Mux9/1 -> [voltage_9]
  Subsystem/35(x_voltage_per_switching_state8) -> Mux9/3
  Data Type Conversion43/1 -> Delay54/1
  Delay55/1 -> y_voltage_per_switching_state_10/1, y_voltage_per_switching_state_AXI_10/1
  Demux10/2 -> Data Type Conversion45/1
  Delay53/1 -> q_voltage_per_switching_state_10/1, q_voltage_per_switching_state_AXI_10/1
  Demux10/1 -> Data Type Conversion42/1
  Delay54/1 -> x_voltage_per_switching_state_10/1, x_voltage_per_switching_state_AXI_10/1
  Delay52/1 -> d_voltage_per_switching_state_10/1, d_voltage_per_switching_state_AXI_10/1
  Data Type Conversion44/1 -> Delay55/1
  Demux10/3 -> Data Type Conversion43/1
  Demux10/4 -> Data Type Conversion44/1
  Data Type Conversion45/1 -> Delay53/1
  Data Type Conversion42/1 -> Delay52/1
  [voltage_10] -> Demux10/1
  Mux10/1 -> [voltage_10]
  Subsystem/40(y_voltage_per_switching_state9) -> Mux10/4
  Subsystem/39(x_voltage_per_switching_state9) -> Mux10/3
  Subsystem/37(d_voltage_per_switching_state9) -> Mux10/1
  Subsystem/38(q_voltage_per_switching_state9) -> Mux10/2
  Data Type Conversion49/1 -> Delay57/1
  Data Type Conversion46/1 -> Delay56/1
  [voltage_11] -> Demux11/1
  Demux11/3 -> Data Type Conversion47/1
  Demux11/4 -> Data Type Conversion48/1
  Demux11/2 -> Data Type Conversion49/1
  Delay57/1 -> q_voltage_per_switching_state_11/1, q_voltage_per_switching_state_AXI_11/1
  Demux11/1 -> Data Type Conversion46/1
  Delay58/1 -> x_voltage_per_switching_state_11/1, x_voltage_per_switching_state_AXI_11/1
  Delay59/1 -> y_voltage_per_switching_state_11/1, y_voltage_per_switching_state_AXI_11/1
  Delay56/1 -> d_voltage_per_switching_state_11/1, d_voltage_per_switching_state_AXI_11/1
  Data Type Conversion47/1 -> Delay58/1
  Data Type Conversion48/1 -> Delay59/1
  Mux11/1 -> [voltage_11]
  Subsystem/43(x_voltage_per_switching_state10) -> Mux11/3
  Subsystem/41(d_voltage_per_switching_state10) -> Mux11/1
  Subsystem/42(q_voltage_per_switching_state10) -> Mux11/2
  Subsystem/44(y_voltage_per_switching_state10) -> Mux11/4
  Delay62/1 -> x_voltage_per_switching_state_12/1, x_voltage_per_switching_state_AXI_12/1
  Delay61/1 -> q_voltage_per_switching_state_12/1, q_voltage_per_switching_state_AXI_12/1
  Data Type Conversion53/1 -> Delay61/1
  Data Type Conversion50/1 -> Delay60/1
  [voltage_12] -> Demux12/1
  Demux12/3 -> Data Type Conversion51/1
  Demux12/4 -> Data Type Conversion52/1
  Demux12/1 -> Data Type Conversion50/1
  Demux12/2 -> Data Type Conversion53/1
  Delay60/1 -> d_voltage_per_switching_state_12/1, d_voltage_per_switching_state_AXI_12/1
  Data Type Conversion52/1 -> Delay63/1
  Data Type Conversion51/1 -> Delay62/1
  Delay63/1 -> y_voltage_per_switching_state_12/1, y_voltage_per_switching_state_AXI_12/1
  Subsystem/48(y_voltage_per_switching_state11) -> Mux12/4
  Subsystem/46(q_voltage_per_switching_state11) -> Mux12/2
  Subsystem/47(x_voltage_per_switching_state11) -> Mux12/3
  Subsystem/45(d_voltage_per_switching_state11) -> Mux12/1
  Mux12/1 -> [voltage_12]
  Delay67/1 -> y_voltage_per_switching_state_13/1, y_voltage_per_switching_state_AXI_13/1
  Data Type Conversion55/1 -> Delay66/1
  Data Type Conversion56/1 -> Delay67/1
  Demux13/2 -> Data Type Conversion57/1
  Demux13/4 -> Data Type Conversion56/1
  Demux13/1 -> Data Type Conversion54/1
  [voltage_13] -> Demux13/1
  Demux13/3 -> Data Type Conversion55/1
  Delay65/1 -> q_voltage_per_switching_state_13/1, q_voltage_per_switching_state_AXI_13/1
  Data Type Conversion57/1 -> Delay65/1
  Delay64/1 -> d_voltage_per_switching_state_13/1, d_voltage_per_switching_state_AXI_13/1
  Delay66/1 -> x_voltage_per_switching_state_13/1, x_voltage_per_switching_state_AXI_13/1
  Data Type Conversion54/1 -> Delay64/1
  Mux13/1 -> [voltage_13]
  Subsystem/52(y_voltage_per_switching_state12) -> Mux13/4
  Subsystem/50(q_voltage_per_switching_state12) -> Mux13/2
  Subsystem/51(x_voltage_per_switching_state12) -> Mux13/3
  Subsystem/49(d_voltage_per_switching_state12) -> Mux13/1
  [voltage_14] -> Demux14/1
  Demux14/1 -> Data Type Conversion58/1
  Demux14/4 -> Data Type Conversion60/1
  Data Type Conversion60/1 -> Delay71/1
  Demux14/2 -> Data Type Conversion61/1
  Data Type Conversion59/1 -> Delay70/1
  Delay71/1 -> y_voltage_per_switching_state_14/1, y_voltage_per_switching_state_AXI_14/1
  Data Type Conversion58/1 -> Delay68/1
  Delay70/1 -> x_voltage_per_switching_state_14/1, x_voltage_per_switching_state_AXI_14/1
  Delay68/1 -> d_voltage_per_switching_state_14/1, d_voltage_per_switching_state_AXI_14/1
  Data Type Conversion61/1 -> Delay69/1
  Demux14/3 -> Data Type Conversion59/1
  Delay69/1 -> q_voltage_per_switching_state_14/1, q_voltage_per_switching_state_AXI_14/1
  Subsystem/56(y_voltage_per_switching_state13) -> Mux14/4
  Subsystem/53(d_voltage_per_switching_state13) -> Mux14/1
  Subsystem/55(x_voltage_per_switching_state13) -> Mux14/3
  Subsystem/54(q_voltage_per_switching_state13) -> Mux14/2
  Mux14/1 -> [voltage_14]
  Subsystem/57(d_voltage_per_switching_state14) -> Mux15/1
  Subsystem/60(y_voltage_per_switching_state14) -> Mux15/4
  Subsystem/59(x_voltage_per_switching_state14) -> Mux15/3
  Subsystem/58(q_voltage_per_switching_state14) -> Mux15/2
  Mux15/1 -> [voltage_15]
  Data Type Conversion64/1 -> Delay75/1
  Demux15/4 -> Data Type Conversion64/1
  Demux15/1 -> Data Type Conversion62/1
  Data Type Conversion63/1 -> Delay74/1
  Demux15/2 -> Data Type Conversion65/1
  [voltage_15] -> Demux15/1
  Demux15/3 -> Data Type Conversion63/1
  Delay72/1 -> d_voltage_per_switching_state_15/1, d_voltage_per_switching_state_AXI_15/1
  Delay73/1 -> q_voltage_per_switching_state_15/1, q_voltage_per_switching_state_AXI_15/1
  Data Type Conversion65/1 -> Delay73/1
  Delay75/1 -> y_voltage_per_switching_state_15/1, y_voltage_per_switching_state_AXI_15/1
  Data Type Conversion62/1 -> Delay72/1
  Delay74/1 -> x_voltage_per_switching_state_15/1, x_voltage_per_switching_state_AXI_15/1
